simulink model "test"  (R2020a)
settings: Solver=VariableStepAuto  StartTime=0.0  StopTime=30  FixedStep=0.01  RelTol=1e-3
undefined symbols (not defined in the file or in its folder): para_u, para_yaw
settings Model: Creator=45489  LastModifiedBy=45489

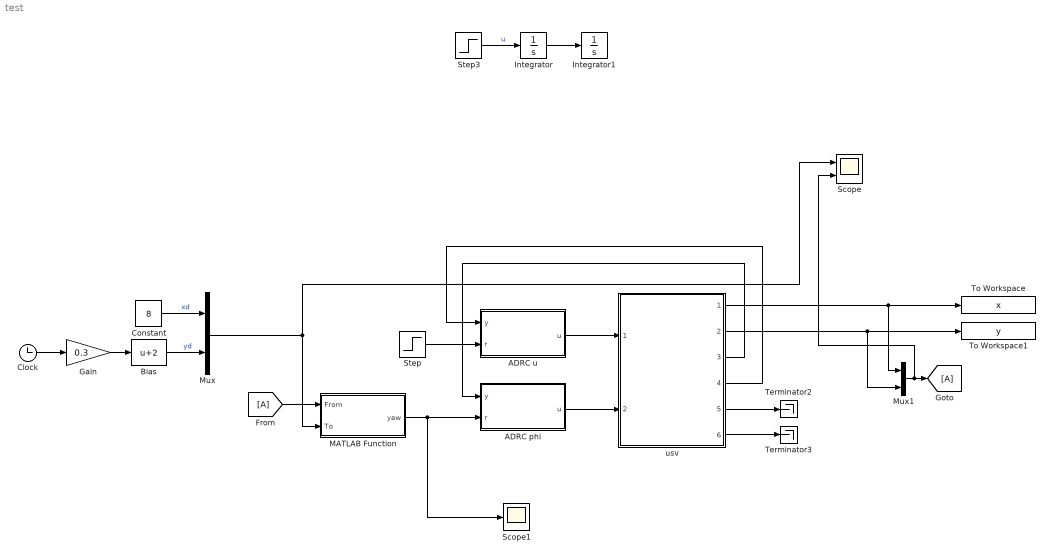
== system test ==
  ADRC phi : Subsystem
  ADRC u : Subsystem
  Bias : Bias  Bias=2
  Clock : Clock
  Constant : Constant  Value=8
  Gain : Gain  Gain=0.3
  Integrator : Integrator
  Integrator1 : Integrator
  MATLAB Function : MATLAB Function  TreatAsAtomicUnit=on
  Mux : Mux  Inputs=2
  Mux1 : Mux  Inputs=2
  Scope : Scope  NumInputPorts=2
  Scope1 : Scope
  Step : Step  After=0.3  SampleTime=0
  Step3 : Step  SampleTime=0
  Terminator2 : Terminator
  Terminator3 : Terminator
  To Workspace : ToWorkspace  VariableName=x  SaveFormat=Timeseries  SampleTime=-1
  To Workspace1 : ToWorkspace  VariableName=y  SaveFormat=Timeseries  SampleTime=-1
  usv : Subsystem  ReferencedSubsystem=USV_Model
  wires:
  Integrator/1 -> Integrator1/1
  Step3/1 -> Integrator/1  "u"
  usv/3 -> ADRC phi/1(y)
  usv/2 -> To Workspace1/1, Mux1/2
  usv/4 -> ADRC u/1(y)
  usv/1 -> Mux1/1, To Workspace/1
  ADRC phi/1(u) -> usv/2
  usv/5 -> Terminator2/1
  Step/1 -> ADRC u/2(r)
  usv/6 -> Terminator3/1
  MATLAB Function/1(yaw) -> Scope1/1, ADRC phi/2(r)
  ADRC u/1(u) -> usv/1
  Clock/1 -> Gain/1
  Gain/1 -> Bias/1
  Constant/1 -> Mux/1  "xd"
  Mux/1 -> MATLAB Function/2(To), Scope/1
  Mux1/1 -> Scope/2, [A]
  [A] -> MATLAB Function/1(From)
  Bias/1 -> Mux/2  "yd"

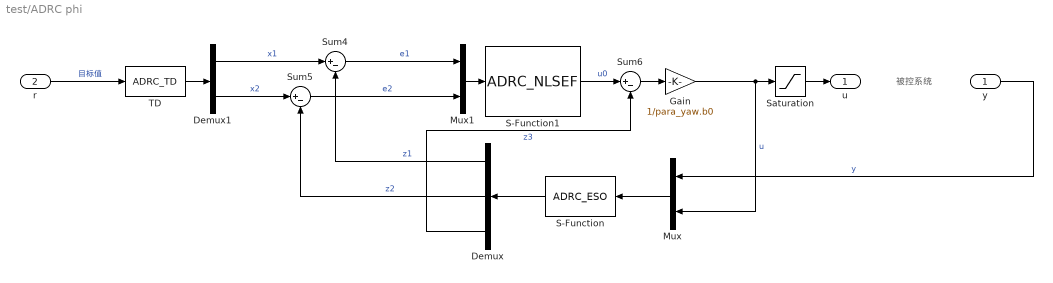
== system test/ADRC phi ==
  note: 被控系统
  y : Inport
  r : Inport  Port=2
  Demux : Demux  Outputs=3
  Demux1 : Demux  Outputs=2
  Gain : Gain  Gain=1/para_yaw.b0
  Mux : Mux  Inputs=2
  Mux1 : Mux  Inputs=2
  S-Function : S-Function  FunctionName=ADRC_ESO  Parameters=para_yaw  SFunctionDeploymentMode=off  EnableBusSupport=off
  S-Function1 : S-Function  FunctionName=ADRC_NLSEF  Parameters=para_yaw  SFunctionDeploymentMode=off  EnableBusSupport=off
  Saturation : Saturate  UpperLimit=50  LowerLimit=-50
  Sum4 : Sum  Inputs=|+-
  Sum5 : Sum  Inputs=|+-
  Sum6 : Sum  Inputs=|+-
  TD : S-Function  FunctionName=ADRC_TD  Parameters=para_yaw  SFunctionDeploymentMode=off  EnableBusSupport=off
  u : Outport
  wires:
  y/1 -> Mux/1  "y"
  TD/1 -> Demux1/1
  Gain/1 -> Saturation/1, Mux/2  "u"
  Mux/1 -> S-Function/1
  S-Function/1 -> Demux/1
  Demux1/1 -> Sum4/1  "x1"
  Sum6/1 -> Gain/1
  Demux1/2 -> Sum5/1  "x2"
  Demux/2 -> Sum5/2  "z2"
  r/1 -> TD/1  "目标值"
  Sum4/1 -> Mux1/1  "e1"
  Demux/3 -> Sum6/2  "z3"
  Demux/1 -> Sum4/2  "z1"
  Mux1/1 -> S-Function1/1
  Sum5/1 -> Mux1/2  "e2"
  S-Function1/1 -> Sum6/1  "u0"
  Saturation/1 -> u/1

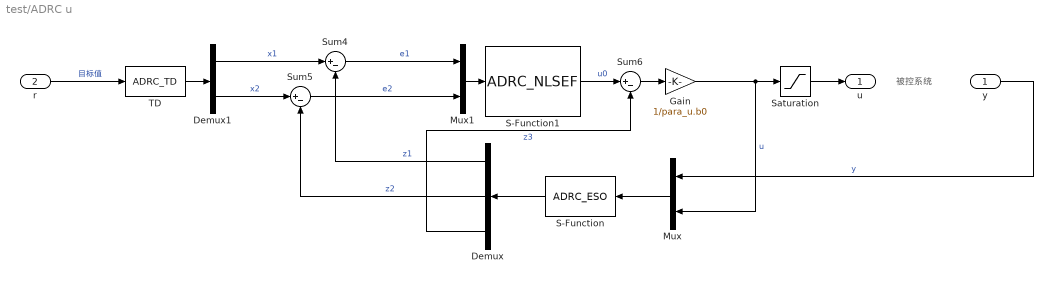
== system test/ADRC u ==
  note: 被控系统
  y : Inport
  r : Inport  Port=2
  Demux : Demux  Outputs=3
  Demux1 : Demux  Outputs=2
  Gain : Gain  Gain=1/para_u.b0
  Mux : Mux  Inputs=2
  Mux1 : Mux  Inputs=2
  S-Function : S-Function  FunctionName=ADRC_ESO  Parameters=para_u  SFunctionDeploymentMode=off  EnableBusSupport=off
  S-Function1 : S-Function  FunctionName=ADRC_NLSEF  Parameters=para_u  SFunctionDeploymentMode=off  EnableBusSupport=off
  Saturation : Saturate  UpperLimit=100  LowerLimit=0
  Sum4 : Sum  Inputs=|+-
  Sum5 : Sum  Inputs=|+-
  Sum6 : Sum  Inputs=|+-
  TD : S-Function  FunctionName=ADRC_TD  Parameters=para_u  SFunctionDeploymentMode=off  EnableBusSupport=off
  u : Outport
  wires:
  y/1 -> Mux/1  "y"
  TD/1 -> Demux1/1
  Gain/1 -> Saturation/1, Mux/2  "u"
  Mux/1 -> S-Function/1
  S-Function/1 -> Demux/1
  Demux1/1 -> Sum4/1  "x1"
  Sum6/1 -> Gain/1
  Demux1/2 -> Sum5/1  "x2"
  Demux/2 -> Sum5/2  "z2"
  r/1 -> TD/1  "目标值"
  Sum4/1 -> Mux1/1  "e1"
  Demux/3 -> Sum6/2  "z3"
  Demux/1 -> Sum4/2  "z1"
  Mux1/1 -> S-Function1/1
  Sum5/1 -> Mux1/2  "e2"
  S-Function1/1 -> Sum6/1  "u0"
  Saturation/1 -> u/1

== matlab function test/MATLAB Function ==
  data: From input; yaw output; To input
function yaw = desierd_yaw(From, To)
% generate path
% t=[0:0.1:30];
% x=8*ones(size(t));
% y=t+2;
% horzcat(x',y')

% closest point


% calculate yaw
d=To-From;
yaw=0;
if d(1)>0
    yaw=atan(d(2)/d(1));
elseif d(1)<=0 && d(2) >0
    yaw=pi+atan(d(2)/d(1));
elseif d(1)<=0 && d(2)<=0
    yaw=-pi+atan(d(2)/d(1));
end
